simulink model "sldvdemo_debounce_adapted_PP"  (R2017b)
settings: Solver=FixedStepDiscrete  StartTime=0.0  StopTime=10.0  FixedStep=0.01  RelTol=1e-3  EnableMultiTasking=on
model workspace (MAT data in the model file):
  already_pp = 1
  compositionalMap.analysisNames = {'sldvdemo_debounce_adapted_PP'}
  compositionalMap.compositionalOptions = {{''}}
  compositionalMap.selectedOptions = 1
  nodeNameToBlockNameMap = containers.Map
  nodeNameToBlockNameMap.serialization.keys = {'A_1', 'A_equal__equal__gt_B_1', 'Assumption_1', 'B_1', 'Constant1_1', 'Constant_1', 'In1_1', 'LogicalOperator1_1', 'LogicalOperator_1', 'RelationalOperator1_1', 'RelationalOperator_1', 'Sum_1', 'Switch_1', 'UnitDelay1_1', 'UnitDelay2_1', 'UnitDelay3_1', 'UnitDelay4_1', 'UnitDelay5_1', 'UnitDelay_1', 'VerifyTrueOutput_310_000', 'debounce_1', 'debounced_1', 'implies_1', 'implies_325_000', 'input_1', 'output_1', 'raw_1', 'sldvdemo_debounce_adapted_PP', 'viewdvc_391_000'}
  nodeNameToBlockNameMap.serialization.values = {'sldvdemo_debounce_adapted_PP/VerifyTrueOutput/implies/A', 'sldvdemo_debounce_adapted_PP/VerifyTrueOutput/implies/A_equal__equal__gt_B', 'sldvdemo_debounce_adapted_PP/Assumption', 'sldvdemo_debounce_adapted_PP/VerifyTrueOutput/implies/B', 'sldvdemo_debounce_adapted_PP/Constant1', 'sldvdemo_debounce_adapted_PP/Constant', 'sldvdemo_debounce_adapted_PP/Assumption/viewdvc/In1', 'sldvdemo_debounce_adapted_PP/VerifyTrueOutput/implies/LogicalOperator1', 'sldvdemo_debounce_adapted_PP/VerifyTrueOutput/implies/LogicalOperator', 'sldvdemo_debounce_adapted_PP/VerifyTrueOutput/RelationalOperator1', 'sldvdemo_debounce_adapted_PP/VerifyTrueOutput/RelationalOperator', 'sldvdemo_debounce_adapted_PP/VerifyTrueOutput/Sum', 'sldvdemo_debounce_adapted_PP/Switch', 'sldvdemo_debounce_adapted_PP/VerifyTrueOutput/UnitDelay1', 'sldvdemo_debounce_adapted_PP/VerifyTrueOutput/UnitDelay2', 'sldvdemo_debounce_adapted_PP/VerifyTrueOutput/UnitDelay3', 'sldvdemo_debounce_adapted_PP/VerifyTrueOutput/UnitDelay4', 'sldvdemo_debounce_adapted_PP/VerifyTrueOutput/UnitDelay5', 'sldvdemo_debounce_adapted_PP/VerifyTrueOutput/UnitDelay', 'sldvdemo_debounce_adapted_PP/VerifyTrueOutput/Assertion', 'sldvdemo_debounce_adapted_PP/debounce', 'sldvdemo_debounce_adapted_PP/debounced', 'sldvdemo_debounce_adapted_PP/VerifyTrueOutput/implies', 'sldvdemo_debounce_adapted_PP/VerifyTrueOutput/implies', 'sldvdemo_debounce_adapted_PP/VerifyTrueOutput/input', 'sldvdemo_debounce_adapted_PP/VerifyTrueOutput/output', 'sldvdemo_debounce_adapted_PP/raw', 'sldvdemo_debounce_adapted_PP', 'sldvdemo_debounce_adapted_PP/Assumption/viewdvc'}
  nodeNameToBlockNameMap.serialization.uniformity = 1
  nodeNameToBlockNameMap.serialization.keyType = 'char'
  nodeNameToBlockNameMap.serialization.valueType = 'char'
  verificationResults.analysisResults{1}.top = 'sldvdemo_debounce_adapted_PP'
  verificationResults.analysisResults{1}.abstract = ''
  verificationResults.analysisResults{1}.concrete = 'implies_325_000,debounce_95_Node,debounce_95_EntryAction,debounce_95_DefaultTrans_Node,debounce_363_000,VerifyTrueOutput_310_000,To_on_96_OuterTrans_Node,To_on_96_Node,To_on_96_ExitAction,To_on_96_EntryAction,To_on_96_DuringAction,To_off_98_OuterTrans_Node,To_off_98_Node,To_off_98_ExitAction,To_off_98_EntryAction,To_off_98_DuringAction,On_99_OuterTrans_Node,On_99_Node,On_99_ExitAction,On_99_EntryAction,Off_97_OuterTrans_Node,Off_97_Node,Off_97_ExitAction,Off_97_EntryAction'
  verificationResults.analysisResults{1}.assumptions = ''
  verificationResults.analysisResults{1}.properties{1}.propertyName = 'VerifyTrueOutput_310_000[l483c36].Assertion_313_000'
  verificationResults.analysisResults{1}.properties{1}.answer = 'SAFE'
  verificationResults.analysisResults{1}.properties{1}.originPath = 'sldvdemo_debounce_adapted_PP/VerifyTrueOutput/Assertion'
  verificationResults.analysisResults{1}.properties{1}.propertyType = 'localProperty'
  verificationResults.sampleTime = 0.01
undefined symbols (not defined in the file): sldvsubsys
Description:
  | Property Proving with an Assumption Block
  | 
  | This example shows how to perform a Simulink Design Verifier property proof using a
  | Proof Assumption block.
settings Model: Creator=The MathWorks, Inc.  LastModifiedBy=hbourbou
settings SolverCC: InsertRTBMode=Auto
settings DataIOCC: LimitDataPoints=on  SaveFormat=Array
settings OptimizationCC: DefaultParameterBehavior=Inlined  ExpressionDepthLimit=2147483647  InitFltsAndDblsToZero=on  EfficientMapNaN2IntZero=off  LifeSpan=inf
settings DebuggingCC: AlgebraicLoopMsg=error  SaveWithParameterizedLinksMsg=none  UnderspecifiedInitializationDetection=Classic  MergeDetectMultiDrivingBlocksExec=none  SignalResolutionControl=TryResolveAllWithWarning  SolverPrmCheckMsg=warning  FcnCallInpInsideContextMsg=warning  StateNameClashWarn=warning  StrictBusMsg=Warning  SFUnexpectedBacktrackingDiag=warning  SFNoUnconditionalDefaultTransitionDiag=warning  SFExecutionAtInitializationDiag=none
settings HardwareCC: ProdBitPerPointer=32  ProdBitPerSizeT=32  ProdBitPerPtrDiffT=32  ProdLargestAtomicFloat=None  ProdIntDivRoundTo=Undefined  ProdEndianess=Unspecified  ProdWordSize=32  ProdHWDeviceType=32-bit Generic
settings ModelReferenceCC: PropagateSignalLabelsOutOfModel=off
settings SFSimCC: SimParseCustomCode=off
settings CodeAppCC: StateflowObjectComments=on
settings GRTTargetCC: TargetFcnLib=ansi_tfl_tmw.mat  TargetLangStandard=C89/C90 (ANSI)  GeneratePreprocessorConditionals=Disable all  CombineOutputUpdateFcns=off  GRTInterface=on
settings ConfigComp: DVMode=PropertyProving  DVMaxProcessTime=1200  DVMakeOutputFilesUnique=off  DVParameters=on  DVModelCoverageObjectives=MCDC  DVMaxTestCaseSteps=500  DVTestSuiteOptimization=CombinedObjectives  DVAssertions=EnableAll  DVProofAssumptions=EnableAll  DVDetectActiveLogic=on  DVDetectFloatOverflow=off  DVModelReferenceHarness=on

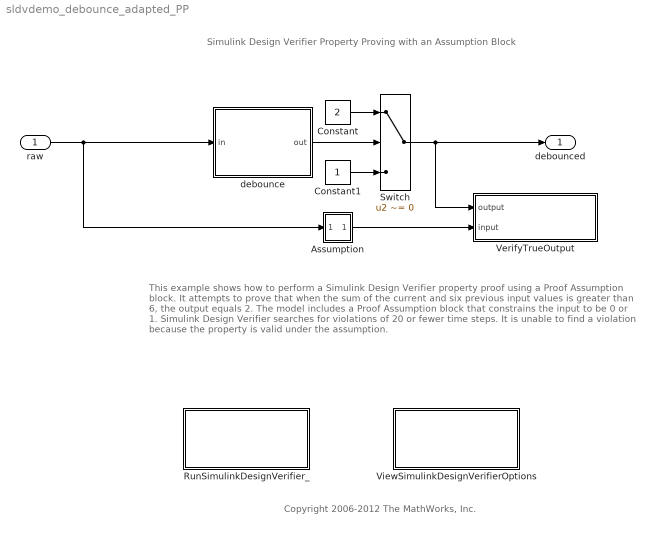
== system sldvdemo_debounce_adapted_PP ==
  note: Copyright 2006-2012 The MathWorks, Inc.
  note: This example shows how to perform a Simulink Design Verifier property proof using a
      | Proof Assumption block. It attempts to prove that when the sum of the current and six
      | previous input values is greater than 6, the output equals 2. The model includes a
      | Proof Assumption block that constrains the input to be 0 or 1.
      |
      | Simulink Design Verifier searches for violations of 20 or fewer time steps.  It is unable
      | to find a violation because the property is valid under the assumption.
  note: Simulink Design Verifier
      | Property Proving with an Assumption Block
  raw : Inport  OutDataTypeStr=double
  Assumption : Subsystem  AncestorBlock=sldvlib/Objectives and Constraints/Assumption  TreatAsAtomicUnit=on  mask(Design Verifier Assumption){enabled=on, customAVTBlockType=Assumption, intervals={0, 1}, initial=off, dispValues=on, outEnabled=on}
      mask prompts: enabled "Sldv:shared:sldvlibrary:Enable"; customAVTBlockType "Sldv:shared:sldvlibrary:Type"; intervals "Sldv:shared:sldvlibrary:Values"; initial "Sldv:shared:sldvlibrary:Initial"; dispValues "Sldv:shared:sldvlibrary:DispValues"; outEnabled "Sldv:shared:sldvlibrary:PassThrough"
      mask help: Sldv:shared:sldvlibrary:AssumptionDesc
      mask init:
      | customAVTParams = customAVTBlock(gcb, 'update_from_mask', intervals);
      settings: AttributesFormatString=%<intervals>
      mask Help: helpview(fullfile(docroot,'toolbox','sldv','sldv.map'),'proofassumption')
      mask TypeOptions customAVTBlockType: Sldv:shared:sldvlibrary:ObjectiveTypeTestCondition | Sldv:shared:sldvlibrary:ObjectiveTypeAssumption
      mask Callback dispValues: customAVTBlock(gcb,'updateDisp');
      mask Display: image(imread('sldvicon_a_normal.png','BackGroundColor',[1 1 1]),[3 3 19 20]); hide_arrows(true);
  Constant : Constant  Value=2  OutDataTypeStr=uint8
  Constant1 : Constant  OutDataTypeStr=uint8
  RunSimulinkDesignVerifier_ : Subsystem  AncestorBlock=sldvdemowidgets/Run Simulink Design Verifier  TreatAsAtomicUnit=on
      settings: OpenFcn=sldvdemo_helper('run',gcbh);
      mask Display: disp('Run \n (double-click)')
  Switch : Switch  Criteria=u2 ~= 0
  VerifyTrueOutput : Subsystem  Tag=VerificationSubsystem  DisableCoverage=on  LoadFcn=sldvsubsys('check')  TreatAsAtomicUnit=on  SimViewingDevice=on  mask(VerificationSubsystem){}
      mask init:
      | sldvsubsys('maskInit');
      settings: CopyFcn=sldvsubsys('copy');
      settings: PreSaveFcn=|
      | set_param(gcb,'SimViewingDevice','on');
      | sldvsubsys('check');
      mask Display: image(imread('sldvicon_versubsys.png','BackGroundColor',[1 1 1]),'center');
  ViewSimulinkDesignVerifierOptions : Subsystem  AncestorBlock=sldvdemowidgets/View Simulink Design Verifier Options  TreatAsAtomicUnit=on
      settings: OpenFcn=sldvdemo_helper('showopts',gcbh);
      mask Display: disp('View Options \n (double-click)')
  debounce : Stateflow chart  TreatAsAtomicUnit=on
  debounced : Outport  OutDataTypeStr=uint8
  wires:
  debounce/1(out) -> Switch/2
  Switch/1 -> debounced/1, VerifyTrueOutput/1(output)
  Constant/1 -> Switch/1
  Constant1/1 -> Switch/3
  Assumption/1(Out1) -> VerifyTrueOutput/2(input)
  raw/1 -> Assumption/1(In1), debounce/1(in)

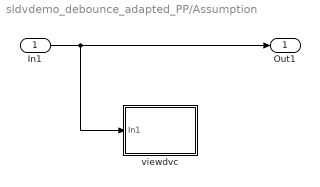
== system sldvdemo_debounce_adapted_PP/Assumption ==
  In1 : Inport
  viewdvc : Subsystem  TreatAsAtomicUnit=on  SimViewingDevice=on  mask(VerificationSubsystem){}
      mask init:
      | sldvsubsys('maskInit');
  Out1 : Outport
  wires:
  In1/1 -> Out1/1, viewdvc/1(In1)

== system sldvdemo_debounce_adapted_PP/RunSimulinkDesignVerifier_ ==

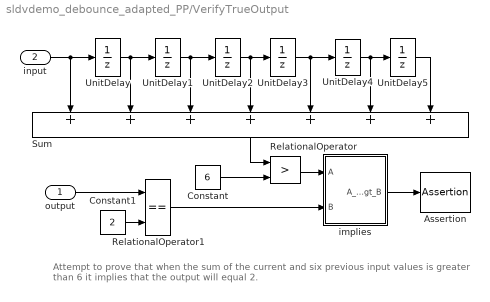
== system sldvdemo_debounce_adapted_PP/VerifyTrueOutput ==
  note: Attempt to prove that when the sum of the current and six previous input
      | values is greater than 6 it implies that the output will equal 2.
  output : Inport
  input : Inport  Port=2
  Assertion : Assertion  StopWhenAssertionFail=off
  Constant : Constant  Value=6  OutDataTypeStr=double
  Constant1 : Constant  Value=2  OutDataTypeStr=uint8
  RelationalOperator : RelationalOperator  Operator=>  OutDataTypeStr=boolean  RndMeth=Nearest
  RelationalOperator1 : RelationalOperator  Operator===  OutDataTypeStr=boolean  RndMeth=Nearest
  Sum : Sum  Inputs=+++++++
  UnitDelay{,1..5} (6 alike) : UnitDelay  SampleTime=-1
  implies : Subsystem  TreatAsAtomicUnit=on
  wires:
  input/1 -> UnitDelay/1, Sum/1
  UnitDelay/1 -> UnitDelay1/1, Sum/2
  UnitDelay1/1 -> UnitDelay2/1, Sum/3
  UnitDelay2/1 -> UnitDelay3/1, Sum/4
  UnitDelay3/1 -> UnitDelay4/1, Sum/5
  UnitDelay4/1 -> Sum/6, UnitDelay5/1
  Sum/1 -> RelationalOperator/1
  Constant/1 -> RelationalOperator/2
  Constant1/1 -> RelationalOperator1/2
  output/1 -> RelationalOperator1/1
  RelationalOperator/1 -> implies/1(A)
  RelationalOperator1/1 -> implies/2(B)
  implies/1(A_equal__equal__gt_B) -> Assertion/1
  UnitDelay5/1 -> Sum/7

== system sldvdemo_debounce_adapted_PP/ViewSimulinkDesignVerifierOptions ==

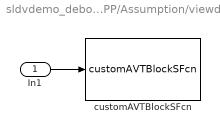
== system sldvdemo_debounce_adapted_PP/Assumption/viewdvc ==
  In1 : Inport
  customAVTBlockSFcn : S-Function  FunctionName=customAVTBlockSFcn  SFunctionDeploymentMode=off  EnableBusSupport=off
  wires:
  In1/1 -> customAVTBlockSFcn/1

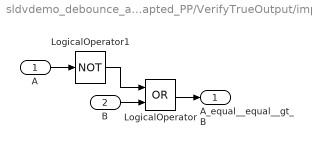
== system sldvdemo_debounce_adapted_PP/VerifyTrueOutput/implies ==
  A : Inport
  B : Inport  Port=2
  LogicalOperator : Logic  Operator=OR  AllPortsSameDT=off  OutDataTypeStr=boolean
  LogicalOperator1 : Logic  Operator=NOT  AllPortsSameDT=off  OutDataTypeStr=boolean
  A_equal__equal__gt_B : Outport
  wires:
  LogicalOperator1/1 -> LogicalOperator/1
  A/1 -> LogicalOperator1/1
  LogicalOperator/1 -> A_equal__equal__gt_B/1
  B/1 -> LogicalOperator/2

== stateflow chart sldvdemo_debounce_adapted_PP/debounce ==
  settings: updateMethod=DISCRETE  sampleTime=0.01
  state To_on
    en: cnt = 0.0;
    du: cnt = cnt + 1;
  state Off
    en: out = false;
  state To_off
    en: cnt = 0.0;
    du: cnt = cnt + 1;
  state On
    en: out = true;
  (default) -> Off
  Off -> To_on : [in==1.0]
  To_on -> Off [order 1] : [in==0.0]
  To_off -> Off [order 2] : [cnt == 4.0]
  To_on -> On [order 2] : [cnt == 4.0]
  On -> To_off : [in==0.0]
  To_off -> On [order 1] : [in==1.0]
  data: in input double; out output boolean; cnt local double
